simulink model "test_atmosphere"  (R2014b)
settings: Solver=ode45  StartTime=0.0  StopTime=10.0  RelTol=1e-3
undefined symbols (not defined in the file or in its folder): TestInputs
libraries: simulink_need_slupdate x10, simulink x2
settings Model: Creator=gnc  LastModifiedBy=mstewart
settings DebuggingCC: UnderspecifiedInitializationDetection=Classic  MergeDetectMultiDrivingBlocksExec=none  SolverPrmCheckMsg=none

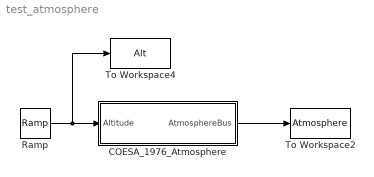
== system test_atmosphere ==
  COESA_1976_Atmosphere : Subsystem  mask(COESA 1976 U.S. Standard Atmosphere){}
      mask help:
      | Committee on Extension to the Standard Atmosphere (COESA) U.S. 1976 Atmosphere Model
      |
      | Computes the atmospheric values of a given geometric  altitude based on the 1976
      | U.S. Standard Atmosphere Model.  This model is valid between -5 km and 1000 km
      | (-16,404 ft and 3,280,840 ft).  Use of this block requires the associated .mat file
      | 'COESA_1976.mat'.
      |
      | Inputs:
      |        Altitude	  [m]   Geometric Altitude
      |
      | Outputs:
      |   CoesaBus
      |
      |        SIGNAL NAME          UNITS       DESCRIPTION
      |        GeometricAlt         [m]         Geometric Altitude
      |        GeopotentialAlt      [m]         Geopotential Altitude
      |        Temp_Kinetic         [deg K]     Kinetic Temperature
      |        Temp_Molecular       [deg K]     Molecular Temperature
      |        Pressure             [Pa]        Atmospheric Pressure
      |        PPo                  [unitless]  Pressure / Pressure0
      |        Density              [kg/m^3]    Atmospheric Density
      |        RhoRho0              [unitless]  Rho / Rho0
      |        Sound                [m/s]       Speed of sound, Cs
      |        DynamicViscosity     [N-s/m^2]   Dynamic Viscosity, mu
      |        KinematicViscosity   [m^2/s]     Kinematic Viscosity, v
      |        kt                   [W/m-K]     Thermal Conductivity
      |        MeanFreePath         [m]          Mean Free Path
      mask init:
      | load COESA_1976.mat
      | 
      | %% Internal Variables
      | r0    = 6.356766e6;  % [m]       Radius of Earth
      | P0    = 1.013250e5;  % [N/m^2]   Standard Pressure at sea level
      | rho0  = 1.2250;      % [kg/m^3]  Standard Density at sea level
  Ramp : simulink/Sources/Ramp  slope=TestInputs.StateBus.AltDot  start=0  X0=TestInputs.StateBus.Alt
  To Workspace2 : ToWorkspace  VariableName=Atmosphere  SaveFormat=Timeseries  SampleTime=-1
  To Workspace4 : ToWorkspace  VariableName=Alt  SaveFormat=Timeseries  SampleTime=-1
  wires:
  COESA_1976_Atmosphere/1(AtmosphereBus) -> To Workspace2/1
  Ramp/1 -> To Workspace4/1, COESA_1976_Atmosphere/1(Altitude)

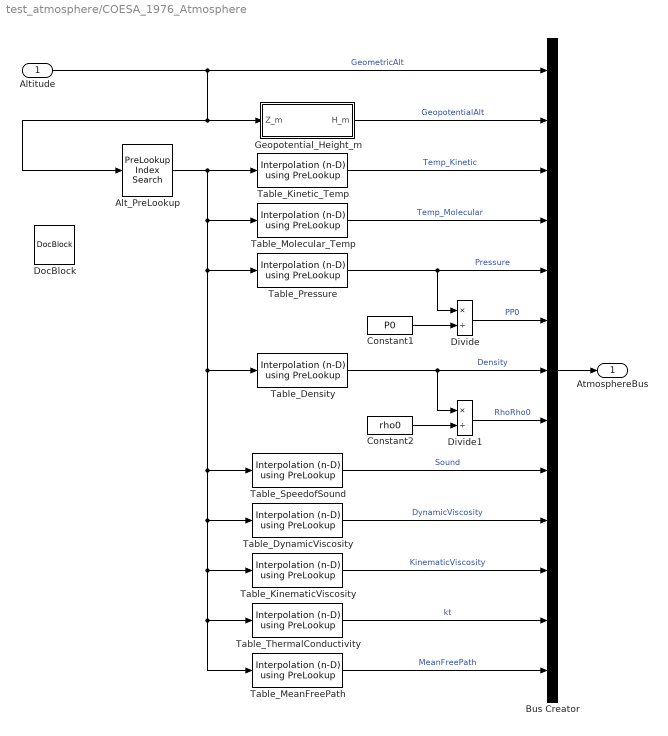
== system test_atmosphere/COESA_1976_Atmosphere ==
  Altitude : Inport
  Alt_PreLookup : simulink_need_slupdate/PreLookup Index Search  bpData=COESA_1976.arrZ  searchMode=Binary Search  cacheBpFlag=off  outputFlag=off  IndexDataType=uint32  extrapMode=Clip to Range  rangeErrorMode=None
  Bus Creator : BusCreator  Inputs=13
  Constant1 : Constant  Value=P0
  Constant2 : Constant  Value=rho0
  Divide : Product  Inputs=*/
  Divide1 : Product  Inputs=*/
  DocBlock : simulink/Model-Wide Utilities/DocBlock  DocumentType=Text
      content=|
      | U.S. Standard Atmosphere, 1976 (COESA 1976)
      |
      | DESCRIPTION
      |    The 1976 U.S. Standard Atmosphere (COESA 1976) is an idealized,
      | steady-state representation of the earth's atmosphere from the surface
      | to 1000 km, { -5 km to 1000 km / -16,404 feet to 3,280,840 feet } as it
      | is assumed to exist in a period of moderate solar activity.
      |
      |   For the lower altitude region (-5 km to 86 km / -16404 ft to 282,152 ft),
      | simple equations can be utilized to compute the desired output values.
      | Here the gases are considered homogeneous.
      |
      |    For the upper atmospheric regions (86 km to 1000 km / 282,152 ft to
      | 3,280,840 ft), these gases undergo dissociation and diffusion.  Since the
      | gases are no longer homogeneous, more sophisticated equations are utilized
      | to correctly model values like the dominant gases' (N2, O, O2, Ar, He, H)
      | number densities.  Since integrations are used in these equations,
      | temperature and pressure computations based on these densities carry large
      | processing times.  To avoid such delays, temperature (both kinetic and
      | molecular), pressure, and air density tables have been generated at 10 m
      | (3313.6 feet) intervals using the DOS executable in Reference 2.
      |
      | NEEDED REFERENCE FILE
      |  Filename: REF_Coesa1976.mat (Generated with 'Build_REF_Coesa1976.m')
      |  Description: Matlab Structure Based on Data Generated by Ref 2.
      |  Form:
      |    REF_Coesa1976       {structure}             COESA 1976
      |        .AllUnits       [1x1 struct]            Units by Parameters
      |        .Description    [1x1 struct]            Description of each .arrXX
      |        .arrZ           [100501x1]  [m]         Geometric Altitude
      |        .arrT_K         [100501x1]  [deg K]     Kinetic Temperature
      |        .arrTm_K        [100501x1]  [deg K]     Molecular Temperature
      |        .arrPress       [100501x1]  [Pa]        Atmospheric Pressure
      |        .arrDensity     [100501x1]  [kg/m^3]    Atmospheric Density
      |        .arrSound       [100501x1]  [m/s]       Speed of Sound
      |        .arrmu          [100501x1]  [N-s/m^2]   Dynamic Viscosity
      |        .arreta         [100501x1]  [m^2/s]     Kinematic Viscosity
      |        .arrkt          [100501x1]  [W/(m-K)]   Coefficient of Thermal
      |                                                 Conductivity
      |
      | SOURCES
      |   Reference 1:
      |    COESA (Committee on Extension to the Standard Atmosphere), U.S.
      |    Standard Atmosphere 1976, U.S. Government Printing Office,
      |    Washington, DC, October 1976.
      |
      |   Reference 2:
      |    "U.S. Standard Atmopsphere 1976"
      |    Online References found through NASA Goddard Space Flight Center
      |
      |    Main Description:
      |      http://nssdc.gsfc.nasa.gov/space/model/atmos/us_standard.html
      |    Turbo Pascal Source Code
      |      http://www.sworld.com.au/steven/space/atmosphere/
      |      Note: This website contains corrections to Reference 1
  Geopotential_Height_m : Subsystem
  Table_Density : simulink_need_slupdate/Interpolation (n-D) using PreLookup  numDimsPopupSelect=1  explicitNumDims=2  table=COESA_1976.arrDensity  interpMethod=Linear  extrapMethod=None - Clip  rangeErrorMode=None  NumSelectionDims=0
  Table_DynamicViscosity : simulink_need_slupdate/Interpolation (n-D) using PreLookup  numDimsPopupSelect=1  explicitNumDims=2  table=COESA_1976.arrmu  interpMethod=Linear  extrapMethod=None - Clip  rangeErrorMode=None  NumSelectionDims=0
  Table_KinematicViscosity : simulink_need_slupdate/Interpolation (n-D) using PreLookup  numDimsPopupSelect=1  explicitNumDims=2  table=COESA_1976.arreta  interpMethod=Linear  extrapMethod=None - Clip  rangeErrorMode=None  NumSelectionDims=0
  Table_Kinetic_Temp : simulink_need_slupdate/Interpolation (n-D) using PreLookup  numDimsPopupSelect=1  explicitNumDims=2  table=COESA_1976.arrT_K  interpMethod=Linear  extrapMethod=None - Clip  rangeErrorMode=None  NumSelectionDims=0
  Table_MeanFreePath : simulink_need_slupdate/Interpolation (n-D) using PreLookup  numDimsPopupSelect=1  explicitNumDims=2  table=COESA_1976.arrL  interpMethod=Linear  extrapMethod=None - Clip  rangeErrorMode=None  NumSelectionDims=0
  Table_Molecular_Temp : simulink_need_slupdate/Interpolation (n-D) using PreLookup  numDimsPopupSelect=1  explicitNumDims=2  table=COESA_1976.arrTm_K  interpMethod=Linear  extrapMethod=None - Clip  rangeErrorMode=None  NumSelectionDims=0
  Table_Pressure : simulink_need_slupdate/Interpolation (n-D) using PreLookup  numDimsPopupSelect=1  explicitNumDims=2  table=COESA_1976.arrPress  interpMethod=Linear  extrapMethod=None - Clip  rangeErrorMode=None  NumSelectionDims=0
  Table_SpeedofSound : simulink_need_slupdate/Interpolation (n-D) using PreLookup  numDimsPopupSelect=1  explicitNumDims=2  table=COESA_1976.arrSound  interpMethod=Linear  extrapMethod=None - Clip  rangeErrorMode=None  NumSelectionDims=0
  Table_ThermalConductivity : simulink_need_slupdate/Interpolation (n-D) using PreLookup  numDimsPopupSelect=1  explicitNumDims=2  table=COESA_1976.arrkt  interpMethod=Linear  extrapMethod=None - Clip  rangeErrorMode=None  NumSelectionDims=0
  AtmosphereBus : Outport
  wires:
  Alt_PreLookup/1 -> Table_MeanFreePath/1, Table_ThermalConductivity/1, Table_KinematicViscosity/1, Table_DynamicViscosity/1, Table_SpeedofSound/1, Table_Density/1, Table_Pressure/1, Table_Molecular_Temp/1, Table_Kinetic_Temp/1
  Table_ThermalConductivity/1 -> Bus Creator/12  "kt"
  Table_KinematicViscosity/1 -> Bus Creator/11  "KinematicViscosity"
  Table_SpeedofSound/1 -> Bus Creator/9  "Sound"
  Table_MeanFreePath/1 -> Bus Creator/13  "MeanFreePath"
  Bus Creator/1 -> AtmosphereBus/1
  Table_DynamicViscosity/1 -> Bus Creator/10  "DynamicViscosity"
  Divide1/1 -> Bus Creator/8  "RhoRho0"
  Constant2/1 -> Divide1/2
  Constant1/1 -> Divide/2
  Divide/1 -> Bus Creator/6  "PP0"
  Geopotential_Height_m/1(H_m) -> Bus Creator/2  "GeopotentialAlt"
  Altitude/1 -> Alt_PreLookup/1, Geopotential_Height_m/1(Z_m), Bus Creator/1  "GeometricAlt"
  Table_Density/1 -> Divide1/1, Bus Creator/7  "Density"
  Table_Pressure/1 -> Divide/1, Bus Creator/5  "Pressure"
  Table_Molecular_Temp/1 -> Bus Creator/4  "Temp_Molecular"
  Table_Kinetic_Temp/1 -> Bus Creator/3  "Temp_Kinetic"

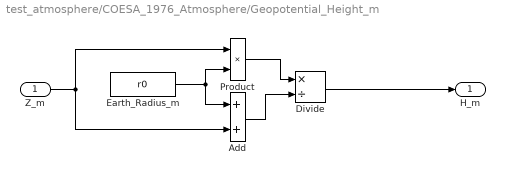
== system test_atmosphere/COESA_1976_Atmosphere/Geopotential_Height_m ==
  Z_m : Inport
  Add : Sum
  Divide : Product  Inputs=*/
  Earth_Radius_m : Constant  Value=r0
  Product : Product  RndMeth=Zero
  H_m : Outport
  wires:
  Earth_Radius_m/1 -> Product/2, Add/1
  Product/1 -> Divide/1
  Add/1 -> Divide/2
  Divide/1 -> H_m/1
  Z_m/1 -> Product/1, Add/2
